simulink model "SingleTrack5states"  (R2018a)
settings: Solver=ode4  StartTime=0.0  StopTime=10  FixedStep=.001  MaxStep=0.001  MinStep=0.0001  RelTol=1e-1
values from neighbouring files (symbols this model uses):
  car = Porsche928    [init.m]
  initBeta = 0    [init.m]
  initR = 0    [init.m]
  initV = 20    [init.m]
settings Model: Creator=efrem  LastModifiedBy=efrem
settings SolverCC: ZeroCrossAlgorithm=Adaptive  AlgebraicLoopSolver=LineSearch
settings DebuggingCC: MaxConsecutiveZCsMsg=none
settings CodeAppCC: StateflowObjectComments=on

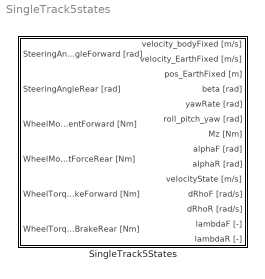
== system SingleTrack5states ==
  SingleTrack5States : Subsystem

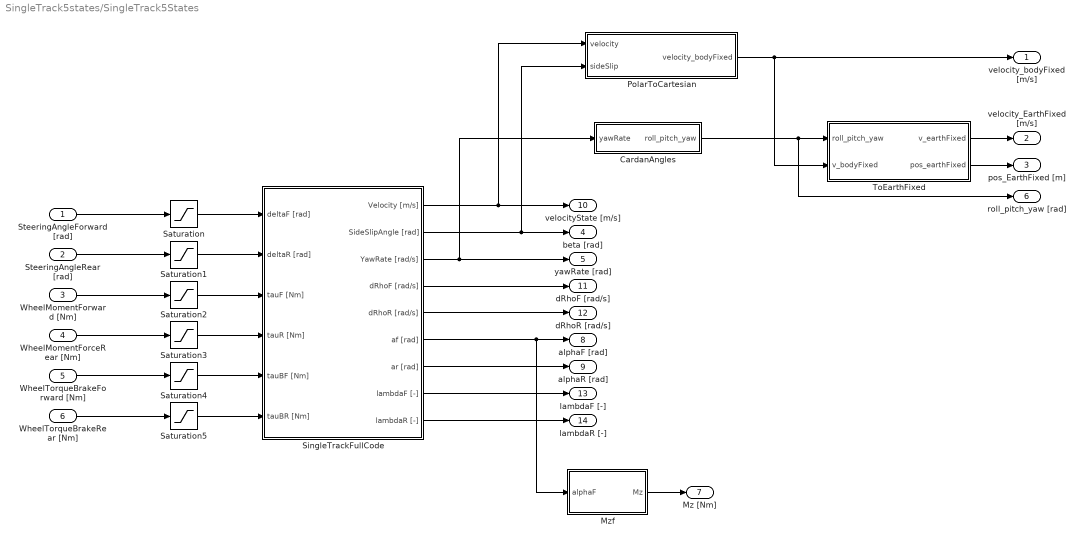
== system SingleTrack5states/SingleTrack5States ==
  SteeringAngleForward [rad] : Inport
  SteeringAngleRear [rad] : Inport  Port=2
  WheelMomentForward [Nm] : Inport  Port=3
  WheelMomentForceRear [Nm] : Inport  Port=4
  WheelTorqueBrakeForward [Nm] : Inport  Port=5
  WheelTorqueBrakeRear [Nm] : Inport  Port=6
  CardanAngles : Subsystem
  Mzf : Subsystem
  PolarToCartesian : Subsystem
  Saturation : Saturate  UpperLimit=pi/3  LowerLimit=-pi/3  ZeroCross=off
  Saturation1 : Saturate  UpperLimit=pi/3  LowerLimit=-pi/3  ZeroCross=off
  Saturation2 : Saturate  UpperLimit=2000  LowerLimit=0  ZeroCross=off
  Saturation3 : Saturate  UpperLimit=2000  LowerLimit=0  ZeroCross=off
  Saturation4 : Saturate  UpperLimit=5000  LowerLimit=0  ZeroCross=off
  Saturation5 : Saturate  UpperLimit=5000  LowerLimit=0  ZeroCross=off
  SingleTrackFullCode : Subsystem
  ToEarthFixed : Subsystem
  velocity_bodyFixed [m/s] : Outport
  velocity_EarthFixed [m/s] : Outport  Port=2
  pos_EarthFixed [m] : Outport  Port=3
  beta [rad] : Outport  Port=4
  yawRate [rad] : Outport  Port=5
  roll_pitch_yaw [rad] : Outport  Port=6
  Mz [Nm] : Outport  Port=7
  alphaF [rad] : Outport  Port=8
  alphaR [rad] : Outport  Port=9
  velocityState [m/s] : Outport  Port=10
  dRhoF [rad/s] : Outport  Port=11
  dRhoR [rad/s] : Outport  Port=12
  lambdaF [-] : Outport  Port=13
  lambdaR [-] : Outport  Port=14
  wires:
  SingleTrackFullCode/3(YawRate [rad/s]) -> CardanAngles/1(yawRate), yawRate [rad]/1
  ToEarthFixed/2(pos_earthFixed) -> pos_EarthFixed [m]/1
  Mzf/1(Mz) -> Mz [Nm]/1
  PolarToCartesian/1(velocity_bodyFixed) -> ToEarthFixed/2(v_bodyFixed), velocity_bodyFixed [m/s]/1
  SingleTrackFullCode/2(SideSlipAngle [rad]) -> PolarToCartesian/2(sideSlip), beta [rad]/1
  ToEarthFixed/1(v_earthFixed) -> velocity_EarthFixed [m/s]/1
  CardanAngles/1(roll_pitch_yaw) -> ToEarthFixed/1(roll_pitch_yaw), roll_pitch_yaw [rad]/1
  SteeringAngleForward [rad]/1 -> Saturation/1
  WheelMomentForward [Nm]/1 -> Saturation2/1
  WheelMomentForceRear [Nm]/1 -> Saturation3/1
  Saturation1/1 -> SingleTrackFullCode/2(deltaR [rad])
  Saturation2/1 -> SingleTrackFullCode/3(tauF [Nm])
  Saturation3/1 -> SingleTrackFullCode/4(tauR [Nm])
  SteeringAngleRear [rad]/1 -> Saturation1/1
  SingleTrackFullCode/1(Velocity [m/s]) -> PolarToCartesian/1(velocity), velocityState [m/s]/1
  WheelTorqueBrakeForward [Nm]/1 -> Saturation4/1
  WheelTorqueBrakeRear [Nm]/1 -> Saturation5/1
  Saturation/1 -> SingleTrackFullCode/1(deltaF [rad])
  Saturation4/1 -> SingleTrackFullCode/5(tauBF [Nm])
  Saturation5/1 -> SingleTrackFullCode/6(tauBR [Nm])
  SingleTrackFullCode/4(dRhoF [rad/s]) -> dRhoF [rad/s]/1
  SingleTrackFullCode/5(dRhoR [rad/s]) -> dRhoR [rad/s]/1
  SingleTrackFullCode/6(af [rad]) -> Mzf/1(alphaF), alphaF [rad]/1
  SingleTrackFullCode/7(ar [rad]) -> alphaR [rad]/1
  SingleTrackFullCode/8(lambdaF [-]) -> lambdaF [-]/1
  SingleTrackFullCode/9(lambdaR [-]) -> lambdaR [-]/1

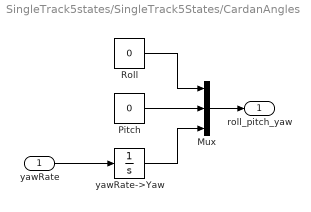
== system SingleTrack5states/SingleTrack5States/CardanAngles ==
  yawRate : Inport
  Mux : Mux  Inputs=3
  Pitch : Constant  Value=0
  Roll : Constant  Value=0
  yawRate->Yaw : Integrator
  roll_pitch_yaw : Outport
  wires:
  Pitch/1 -> Mux/2
  Roll/1 -> Mux/1
  Mux/1 -> roll_pitch_yaw/1
  yawRate->Yaw/1 -> Mux/3
  yawRate/1 -> yawRate->Yaw/1

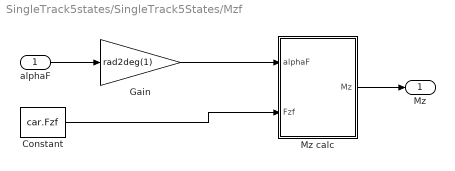
== system SingleTrack5states/SingleTrack5States/Mzf ==
  alphaF : Inport
  Constant : Constant  Value=car.Fzf
  Gain : Gain  Gain=rad2deg(1)
  Mz calc : MATLAB Function  TreatAsAtomicUnit=on
  Mz : Outport
  wires:
  Mz calc/1(Mz) -> Mz/1
  alphaF/1 -> Gain/1
  Constant/1 -> Mz calc/2(Fzf)
  Gain/1 -> Mz calc/1(alphaF)

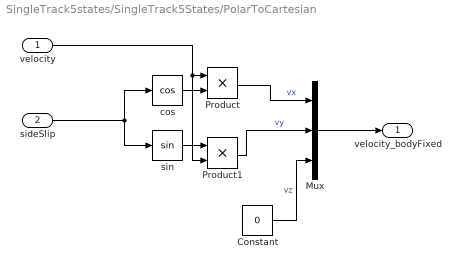
== system SingleTrack5states/SingleTrack5States/PolarToCartesian ==
  velocity : Inport
  sideSlip : Inport  Port=2
  Constant : Constant  Value=0
  Mux : Mux  Inputs=3
  Product : Product
  Product1 : Product
  cos : Trigonometry  Operator=cos
  sin : Trigonometry
  velocity_bodyFixed : Outport
  wires:
  Product/1 -> Mux/1  "vx"
  velocity/1 -> Product/1, Product1/2
  sin/1 -> Product1/1
  sideSlip/1 -> cos/1, sin/1
  Product1/1 -> Mux/2  "vy"
  cos/1 -> Product/2
  Constant/1 -> Mux/3  "vz"
  Mux/1 -> velocity_bodyFixed/1

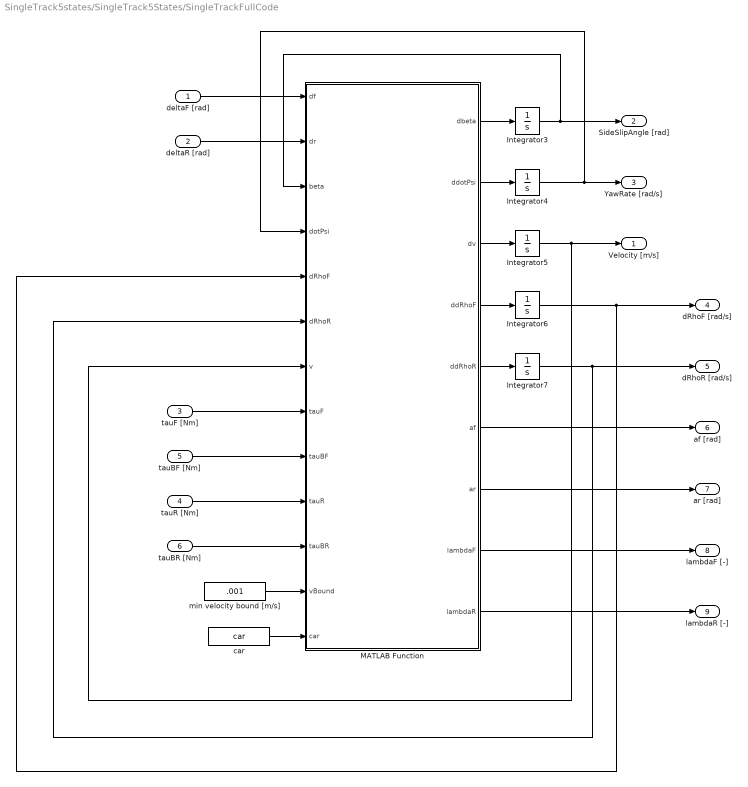
== system SingleTrack5states/SingleTrack5States/SingleTrackFullCode ==
  deltaF [rad] : Inport
  deltaR [rad] : Inport  Port=2
  tauF [Nm] : Inport  Port=3
  tauR [Nm] : Inport  Port=4
  tauBF [Nm] : Inport  Port=5
  tauBR [Nm] : Inport  Port=6
  Integrator3 : Integrator  InitialCondition=initBeta  UpperSaturationLimit=pi/2  LowerSaturationLimit=-pi/2  ZeroCross=off
  Integrator4 : Integrator  InitialCondition=initR  UpperSaturationLimit=pi/2  LowerSaturationLimit=-pi/2  ZeroCross=off
  Integrator5 : Integrator  InitialCondition=initV  UpperSaturationLimit=pi/2  LowerSaturationLimit=-pi/2  ZeroCross=off
  Integrator6 : Integrator  InitialCondition=initV/car.RF  UpperSaturationLimit=pi/2  LowerSaturationLimit=-pi/2  ZeroCross=off
  Integrator7 : Integrator  InitialCondition=initV/car.RR  UpperSaturationLimit=pi/2  LowerSaturationLimit=-pi/2  ZeroCross=off
  MATLAB Function : MATLAB Function  TreatAsAtomicUnit=on
  car : Constant  Value=car  OutDataTypeStr=Bus: car_bus
  min velocity bound [m/s] : Constant  Value=.001
  Velocity [m/s] : Outport
  SideSlipAngle [rad] : Outport  Port=2
  YawRate [rad/s] : Outport  Port=3
  dRhoF [rad/s] : Outport  Port=4
  dRhoR [rad/s] : Outport  Port=5
  af [rad] : Outport  Port=6
  ar [rad] : Outport  Port=7
  lambdaF [-] : Outport  Port=8
  lambdaR [-] : Outport  Port=9
  wires:
  deltaF [rad]/1 -> MATLAB Function/1(df)
  deltaR [rad]/1 -> MATLAB Function/2(dr)
  tauF [Nm]/1 -> MATLAB Function/8(tauF)
  tauR [Nm]/1 -> MATLAB Function/10(tauR)
  car/1 -> MATLAB Function/13(car)
  min velocity bound [m/s]/1 -> MATLAB Function/12(vBound)
  MATLAB Function/1(dbeta) -> Integrator3/1
  Integrator3/1 -> SideSlipAngle [rad]/1, MATLAB Function/3(beta)
  MATLAB Function/2(ddotPsi) -> Integrator4/1
  Integrator4/1 -> YawRate [rad/s]/1, MATLAB Function/4(dotPsi)
  MATLAB Function/3(dv) -> Integrator5/1
  Integrator5/1 -> MATLAB Function/7(v), Velocity [m/s]/1
  MATLAB Function/4(ddRhoF) -> Integrator6/1
  MATLAB Function/5(ddRhoR) -> Integrator7/1
  Integrator7/1 -> dRhoR [rad/s]/1, MATLAB Function/6(dRhoR)
  tauBF [Nm]/1 -> MATLAB Function/9(tauBF)
  tauBR [Nm]/1 -> MATLAB Function/11(tauBR)
  MATLAB Function/6(af) -> af [rad]/1
  MATLAB Function/7(ar) -> ar [rad]/1
  Integrator6/1 -> dRhoF [rad/s]/1, MATLAB Function/5(dRhoF)
  MATLAB Function/8(lambdaF) -> lambdaF [-]/1
  MATLAB Function/9(lambdaR) -> lambdaR [-]/1

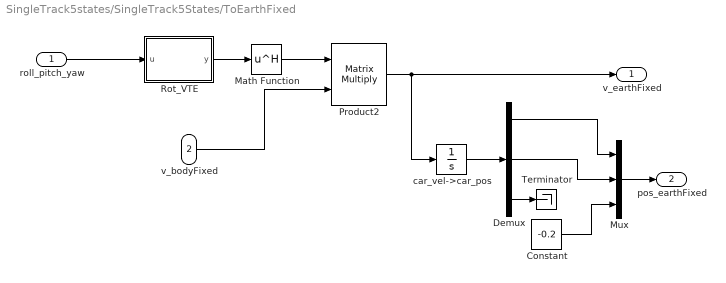
== system SingleTrack5states/SingleTrack5States/ToEarthFixed ==
  roll_pitch_yaw : Inport
  v_bodyFixed : Inport  Port=2
  Constant : Constant  Value=-0.2
  Demux : Demux  Outputs=3
  Math Function : Math  Operator=hermitian  SaturateOnIntegerOverflow=on
  Mux : Mux  Inputs=3
  Product2 : Product  Multiplication=Matrix(*)
  Rot_VTE : MATLAB Function  TreatAsAtomicUnit=on
  Terminator : Terminator
  car_vel->car_pos : Integrator
  v_earthFixed : Outport
  pos_earthFixed : Outport  Port=2
  wires:
  v_bodyFixed/1 -> Product2/2
  Product2/1 -> v_earthFixed/1, car_vel->car_pos/1
  Constant/1 -> Mux/3
  Mux/1 -> pos_earthFixed/1
  car_vel->car_pos/1 -> Demux/1
  Demux/2 -> Mux/2
  Demux/1 -> Mux/1
  Math Function/1 -> Product2/1
  roll_pitch_yaw/1 -> Rot_VTE/1(u)
  Rot_VTE/1(y) -> Math Function/1
  Demux/3 -> Terminator/1

== matlab function SingleTrack5states/SingleTrack5States/ToEarthFixed/Rot_VTE ==
  data: u input; y output
function y = fcn(u)
y = Rot_VTE(u);

== matlab function SingleTrack5states/SingleTrack5States/Mzf/Mz calc ==
  data: alphaF input; Mz output; Fzf input
function Mz = fcn(alphaF, Fzf)
Bz = .15;
Cz = 2.3;
Dz = -.05 * Fzf;
Ez = -10;
Mz = Dz*sin((Cz*atan(Bz*alphaF - Ez*(Bz*alphaF - atan(Bz*alphaF)))));

== matlab function SingleTrack5states/SingleTrack5States/SingleTrackFullCode/MATLAB Function ==
  data: df input; dbeta output; dr input; beta input; dotPsi input; dRhoF input; dRhoR input; v input; tauF input; tauBF input; tauR input; tauBR input; vBound input; car input; ddotPsi output; dv output; ddRhoF output; ddRhoR output; af output; ar output; lambdaF output; lambdaR output
function [dbeta, ddotPsi, dv, ddRhoF, ddRhoR, af, ar, lambdaF, lambdaR]= SingleTrackFullModelFunctionCode(df, dr, beta, dotPsi, dRhoF, dRhoR, v, tauF, tauBF, tauR, tauBR, vBound, car)

    %% parse parameters 
    lf = car.LF;
    lr = car.LR;
    m = car.Mass;
    Fzf = car.Fzf;
    Fzr = car.Fzb;
    Jr = car.JR;
    Jf = car.JF;
    Rr = car.RR;
    Rf = car.RF;
    Iz = car.Iz;
    D = car.Pacejka.D;
    B = car.Pacejka.B;
    C = car.Pacejka.C;
    E = car.Pacejka.E;
    Dx = car.Pacejka.Dx;
    Bx = car.Pacejka.Bx;
    Cx = car.Pacejka.Cx;
    Ex = car.Pacejka.Ex;
    
    %% apply deadzone for the velocity
    if(v < vBound && v >= 0) 
		v = v+vBound;
	elseif (v > -vBound && v <0)
        v = v-vBound;
    end
    
    %% Long. velocities on the wheels
    vxf = v*cos(beta)*cos(df)+(v*sin(beta)+lf*dotPsi)*sin(df);
    vxr = v*cos(beta)*cos(dr)+(v*sin(beta)-lr*dotPsi)*sin(dr);
    
    %% Slip Ratios
    lambdaF = (dRhoF*Rf - vxf)/max(dRhoF*Rf, abs(vxf));
    lambdaR = (dRhoR*Rr - vxr)/max(dRhoR*Rr, abs(vxr));
    
    lambdaF(lambdaF>1) = 1;
    lambdaF(lambdaF<-1) = -1;
    lambdaR(lambdaR>1) = 1;
    lambdaR(lambdaR<-1) = -1;
    
    %% Slip angles
    af = -atan2((v*sin(beta)+lf*dotPsi)*cos(df)-v*cos(beta)*sin(df),...
        abs((v*sin(beta)+lf*dotPsi)*sin(df)+ v*cos(beta)*cos(df)));
    
    ar = -atan2((v*sin(beta)-lr*dotPsi)*cos(dr)-v*cos(beta)*sin(dr),...
        abs((v*sin(beta)-lr*dotPsi)*sin(dr)+ v*cos(beta)*cos(dr)));
    
    %% Pacejka Raw
    af_deg = rad2deg(af); % only in case of my parametrization for degrees
    ar_deg = rad2deg(ar);
    
    Fyf0 = D * Fzf * sin(C * atan(B*af_deg - E*(B*af_deg - atan(B*af_deg))));
    Fyr0 = D * Fzr * sin(C * atan(B*ar_deg - E*(B*ar_deg - atan(B*ar_deg))));

    Fxf0 = Dx * Fzf * sin(Cx * atan(Bx*lambdaF - Ex*(Bx*lambdaF - atan(Bx*lambdaF))));
    Fxr0 = Dx * Fzr * sin(Cx * atan(Bx*lambdaR - Ex*(Bx*lambdaR - atan(Bx*lambdaR))));
    
    %% Traction Ellipse Forward
    
    betaStar = acos(abs(lambdaF)/sqrt(lambdaF^2 + sin(af)^2));

    % friction coefficients
    mu_x_act = Fxf0/Fzf;
    mu_y_act = Fyf0/Fzf;

    mu_x_max = Dx;
    mu_y_max = D;

    mu_x =         1/sqrt((1/mu_x_act)^2 + (tan(betaStar)/mu_y_max)^2 );
    mu_y = tan(betaStar)/sqrt((1/mu_x_max)^2 + (tan(betaStar)/mu_y_act)^2 );

    Fxf = abs(mu_x/mu_x_act)*Fxf0;
    Fyf = abs(mu_y/mu_y_act)*Fyf0;

    if isnan(Fxf)
        Fxf = 0;
    end

    if isnan(Fyf)
        Fyf = 0;
    end

    if Fzf == 0
        Fxf = Fxf0;
        Fyf = Fyf0;
    end
    
    %% Traction Ellipse Rear
    betaStar = acos(abs(lambdaR)/sqrt(lambdaR^2 + sin(ar)^2));

    % friction coefficients
    mu_x_act = Fxr0/Fzr;
    mu_y_act = Fyr0/Fzr;

    mu_x_max = Dx;
    mu_y_max = D;

    mu_x =         1/sqrt((1/mu_x_act)^2 + (tan(betaStar)/mu_y_max)^2 );
    mu_y = tan(betaStar)/sqrt((1/mu_x_max)^2 + (tan(betaStar)/mu_y_act)^2 );

    Fxr = abs(mu_x/mu_x_act)*Fxr0;
    Fyr = abs(mu_y/mu_y_act)*Fyr0;

    if isnan(Fxr)
        Fxr = 0;
    end

    if isnan(Fyr)
        Fyr = 0;
    end

    if Fzr == 0
        Fxr = Fxr0;
        Fyr = Fyr0;
    end
    
    %% Steering angles projection and Dynamics
    
    SAP = [cos(df), -sin(df), cos(dr), -sin(dr);...
        sin(df), cos(df), sin(dr), cos(dr);...
        lf*sin(df), lf*cos(df), -lr*sin(dr), -lr*cos(dr)];

    F = [Fxf; Fyf; Fxr; Fyr];

    RotDyn = [-sin(beta), cos(beta), 0;...
        cos(beta), sin(beta), 0;...
        0, 0, 1];
    
    Dyn = RotDyn * (SAP * F);
    
    % parse to motions
    lat = Dyn(1);
    long = Dyn(2);
    rot = Dyn(3);
    
	%% Body states
    dbeta = - dotPsi + lat/m/v;
    dv = long/m;
    ddotPsi = rot/Iz; 
	
	%% Wheel models
  ddRhoF = (tauF - Rf*Fxf - sign(dRhoF)*tauBF - 5*v- 0.1*v^2)/Jf;
  ddRhoR = (tauR - Rr*Fxr - sign(dRhoR)*tauBR - 5*v- 0.1*v^2)/Jr;
%     ddRhoF = (tauF - Rf*Fxf - sign(dRhoF)*tauBF)/Jf;
%     ddRhoR = (tauR - Rr*Fxr - sign(dRhoR)*tauBR)/Jr;
end
